simulink model "Gateway"  (R2025b)
settings: Solver=FixedStepDiscrete  StartTime=0.0  StopTime=inf  FixedStep=0.01  RelTol=1e-3
StartFcn:
  | qgcMavlinkGatewayVectorStep('reset');
StopFcn:
  | qgcMavlinkGatewayVectorStep('release');
undefined symbols (not defined in the file): CMD_MISSION_CRUISE_SPEED, CMD_MISSION_MAX_ACCELERATION, CMD_MISSION_MAX_JERK
settings Model: DataDictionary=CommandDict.sldd  Creator=89447  LastModifiedBy=89447
settings OptimizationCC: DefaultParameterBehavior=Inlined  EnhancedBackFolding=on  PassReuseOutputArgsAs=Individual arguments  ZeroExternalMemoryAtStartup=off  ZeroInternalMemoryAtStartup=off  MaxStackSize=64  OptimizeBlockOrder=speed  DifferentSizesBufferReuse=on  OptimizationCustomize=off  EfficientTunableParamExpr=on
settings HardwareCC: ProdBitPerLong=64.0  ProdHWDeviceType=Intel->x86-64 (Linux 64)  TargetBitPerLong=64.0  TargetBitPerPointer=64.0  TargetBitPerSizeT=64.0  TargetBitPerPtrDiffT=64.0  TargetLargestAtomicFloat=Float  TargetIntDivRoundTo=Zero  TargetEndianess=LittleEndian  TargetWordSize=64.0  TargetHWDeviceType=Intel->x86-64 (Linux 64)  ProdEqTarget=off
settings ModelReferenceCC: ModelReferenceNumInstancesAllowed=Single
settings SFSimCC: MATLABDynamicMemAlloc=off
settings RTWCC: SystemTargetFile=ert.tlc  HardwareBoard=Robot Operating System 2 (ROS 2)  TLCOptions="-aInlineSetEventsForThisBaseRateFcn=TLC_FALSE -aSuppressMultiTaskScheduler=TLC_FALSE  -aRateBasedStepFcn=0"  TemplateMakefile=ert_default_tmf  Toolchain=Colcon Tools  TargetLang=C++  Description=Embedded Coder
settings CodeAppCC: ForceParamTrailComments=on  IgnoreCustomStorageClasses=off  OperatorAnnotations=on  SimulinkDataObjDesc=on  SFDataObjDesc=on  InsertBlockDesc=on
settings ERTTargetCC: ExtModeTransport=2.0  ExtModeStaticAlloc=on  ExtModeMexFile=ext_xcp  ExtModeIntrfLevel=Level2 - Open  ERTCustomFileTemplate=example_file_process.tlc  TargetLangStandard=C++11 (ISO)  SubcomponentCodeInterfacePackaging=Nonreusable function  SupportContinuousTime=on

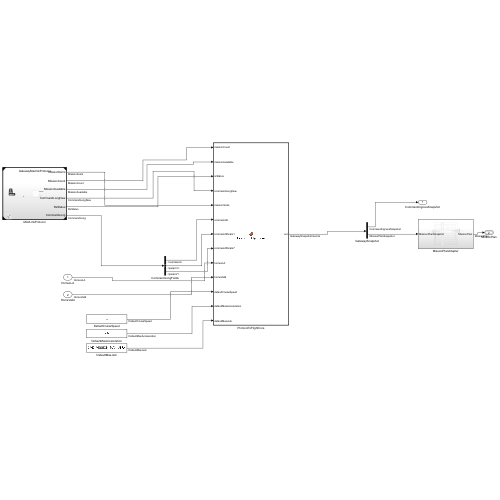
[thumbnail: Simulink's stored preview of the top-level diagram]
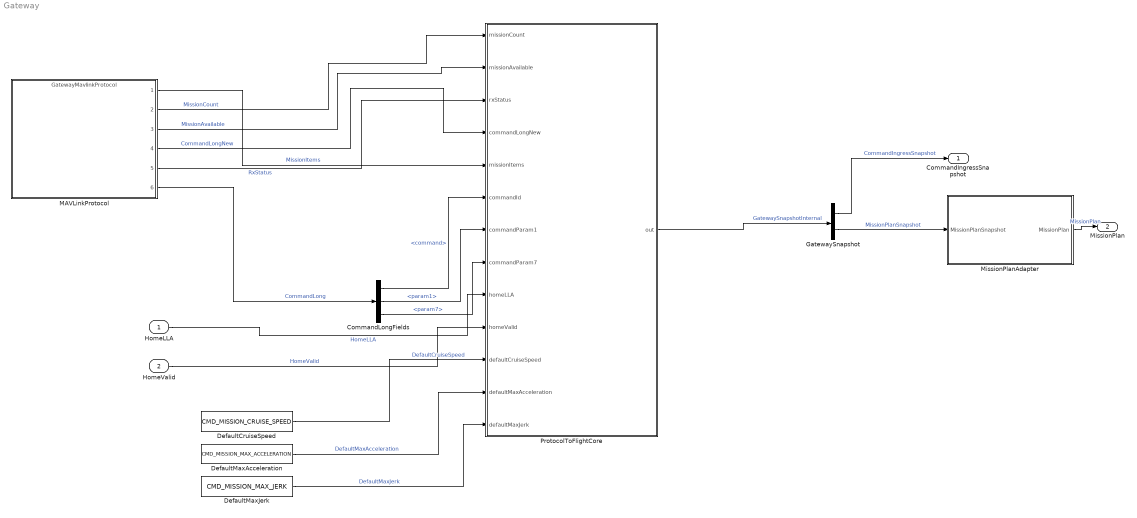
== system Gateway ==
  HomeLLA : Inport  OutDataTypeStr=single  PortDimensions=3
  HomeValid : Inport  Port=2  OutDataTypeStr=boolean  PortDimensions=1
  CommandLongFields : BusSelector  OutputSignals=Payload.command,Payload.param1,Payload.param7
  DefaultCruiseSpeed : Constant  Value=CMD_MISSION_CRUISE_SPEED  OutDataTypeStr=single
  DefaultMaxAcceleration : Constant  Value=CMD_MISSION_MAX_ACCELERATION  OutDataTypeStr=single
  DefaultMaxJerk : Constant  Value=CMD_MISSION_MAX_JERK  OutDataTypeStr=single
  GatewaySnapshot : Demux  Outputs=[17 123]
  MAVLinkProtocol : ModelReference  ModelNameDialog=GatewayMavlinkProtocol  ModelReferenceVersion=10.22
  MissionPlanAdapter : Subsystem
  ProtocolToFlightCore : MATLAB Function  TreatAsAtomicUnit=on
  CommandIngressSnapshot : Outport
  MissionPlan : Outport  Port=2  OutDataTypeStr=Bus: MissionPlanBus
  wires:
  GatewaySnapshot/1 -> CommandIngressSnapshot/1  "CommandIngressSnapshot"
  GatewaySnapshot/2 -> MissionPlanAdapter/1(MissionPlanSnapshot)  "MissionPlanSnapshot"
  MissionPlanAdapter/1(MissionPlan) -> MissionPlan/1  "MissionPlan"
  MAVLinkProtocol/2 -> ProtocolToFlightCore/1(missionCount)  "MissionCount"
  MAVLinkProtocol/3 -> ProtocolToFlightCore/2(missionAvailable)  "MissionAvailable"
  MAVLinkProtocol/4 -> ProtocolToFlightCore/4(commandLongNew)  "CommandLongNew"
  CommandLongFields/1 -> ProtocolToFlightCore/6(commandId)  "<command>"
  CommandLongFields/2 -> ProtocolToFlightCore/7(commandParam1)  "<param1>"
  CommandLongFields/3 -> ProtocolToFlightCore/8(commandParam7)  "<param7>"
  HomeLLA/1 -> ProtocolToFlightCore/9(homeLLA)  "HomeLLA"
  HomeValid/1 -> ProtocolToFlightCore/10(homeValid)  "HomeValid"
  DefaultCruiseSpeed/1 -> ProtocolToFlightCore/11(defaultCruiseSpeed)  "DefaultCruiseSpeed"
  DefaultMaxAcceleration/1 -> ProtocolToFlightCore/12(defaultMaxAcceleration)  "DefaultMaxAcceleration"
  DefaultMaxJerk/1 -> ProtocolToFlightCore/13(defaultMaxJerk)  "DefaultMaxJerk"
  ProtocolToFlightCore/1(out) -> GatewaySnapshot/1  "GatewaySnapshotInternal"
  MAVLinkProtocol/5 -> ProtocolToFlightCore/3(rxStatus)  "RxStatus"
  MAVLinkProtocol/6 -> CommandLongFields/1  "CommandLong"
  MAVLinkProtocol/1 -> ProtocolToFlightCore/5(missionItems)  "MissionItems"

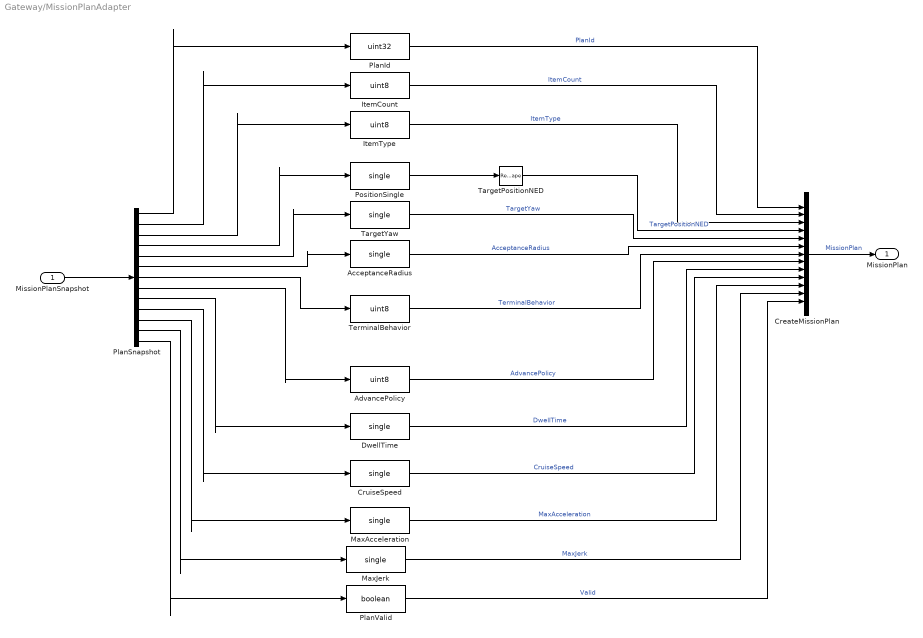
== system Gateway/MissionPlanAdapter ==
  MissionPlanSnapshot : Inport  OutDataTypeStr=double  PortDimensions=123
  AcceptanceRadius : DataTypeConversion  OutDataTypeStr=single
  AdvancePolicy : DataTypeConversion  OutDataTypeStr=uint8
  CreateMissionPlan : BusCreator  Inputs=13  OutDataTypeStr=Bus: MissionPlanBus  NonVirtualBus=on
  CruiseSpeed : DataTypeConversion  OutDataTypeStr=single
  DwellTime : DataTypeConversion  OutDataTypeStr=single
  ItemCount : DataTypeConversion  OutDataTypeStr=uint8
  ItemType : DataTypeConversion  OutDataTypeStr=uint8
  MaxAcceleration : DataTypeConversion  OutDataTypeStr=single
  MaxJerk : DataTypeConversion  OutDataTypeStr=single
  PlanId : DataTypeConversion  OutDataTypeStr=uint32
  PlanSnapshot : Demux  Outputs=[1 1 10 30 10 10 10 10 10 10 10 10 1]
  PlanValid : DataTypeConversion  OutDataTypeStr=boolean
  PositionSingle : DataTypeConversion  OutDataTypeStr=single
  TargetPositionNED : Reshape  OutputDimensionality=Customize  OutputDimensions=[10 3]
  TargetYaw : DataTypeConversion  OutDataTypeStr=single
  TerminalBehavior : DataTypeConversion  OutDataTypeStr=uint8
  MissionPlan : Outport  OutDataTypeStr=Bus: MissionPlanBus
  wires:
  MissionPlanSnapshot/1 -> PlanSnapshot/1
  PlanSnapshot/1 -> PlanId/1
  PlanSnapshot/2 -> ItemCount/1
  PlanSnapshot/3 -> ItemType/1
  PlanSnapshot/4 -> PositionSingle/1
  PositionSingle/1 -> TargetPositionNED/1
  PlanSnapshot/5 -> TargetYaw/1
  PlanSnapshot/6 -> AcceptanceRadius/1
  PlanSnapshot/7 -> TerminalBehavior/1
  PlanSnapshot/8 -> AdvancePolicy/1
  PlanId/1 -> CreateMissionPlan/1  "PlanId"
  ItemCount/1 -> CreateMissionPlan/2  "ItemCount"
  ItemType/1 -> CreateMissionPlan/3  "ItemType"
  TargetPositionNED/1 -> CreateMissionPlan/4  "TargetPositionNED"
  TargetYaw/1 -> CreateMissionPlan/5  "TargetYaw"
  AcceptanceRadius/1 -> CreateMissionPlan/6  "AcceptanceRadius"
  TerminalBehavior/1 -> CreateMissionPlan/7  "TerminalBehavior"
  AdvancePolicy/1 -> CreateMissionPlan/8  "AdvancePolicy"
  CreateMissionPlan/1 -> MissionPlan/1  "MissionPlan"
  PlanSnapshot/13 -> PlanValid/1
  PlanValid/1 -> CreateMissionPlan/13  "Valid"
  PlanSnapshot/9 -> DwellTime/1
  DwellTime/1 -> CreateMissionPlan/9  "DwellTime"
  PlanSnapshot/10 -> CruiseSpeed/1
  CruiseSpeed/1 -> CreateMissionPlan/10  "CruiseSpeed"
  PlanSnapshot/11 -> MaxAcceleration/1
  MaxAcceleration/1 -> CreateMissionPlan/11  "MaxAcceleration"
  PlanSnapshot/12 -> MaxJerk/1
  MaxJerk/1 -> CreateMissionPlan/12  "MaxJerk"

== matlab function Gateway/ProtocolToFlightCore ==
  data: missionCount input; out output; missionAvailable input; rxStatus input; commandLongNew input; missionItems input; commandId input; commandParam1 input; commandParam7 input; homeLLA input; homeValid input; defaultCruiseSpeed input; defaultMaxAcceleration input; defaultMaxJerk input
function out = ProtocolToFlightCore(missionCount, missionAvailable, rxStatus, commandLongNew, missionItems, commandId, commandParam1, commandParam7, homeLLA, homeValid, defaultCruiseSpeed, defaultMaxAcceleration, defaultMaxJerk)
%#codegen
persistent planId lastMissionAvailable rxSequence requestId nowSec lastRxTime linkAge
persistent commanderRequestType commanderRequestValid
persistent missionAction missionRequestValid missionRequestPlanId missionTargetAltitude
if isempty(planId)
    planId = uint32(0);
    lastMissionAvailable = false;
    rxSequence = uint32(0);
    requestId = uint32(0);
    nowSec = single(0);
    lastRxTime = single(0);
    linkAge = single(1000);
    commanderRequestType = uint8(0);
    commanderRequestValid = false;
    missionAction = uint8(0);
    missionRequestValid = false;
    missionRequestPlanId = uint32(0);
    missionTargetAltitude = single(0);
end
out = zeros(1,140);
nowSec = nowSec + single(0.1);
if rxStatus > 0
    rxSequence = rxSequence + uint32(1);
    lastRxTime = nowSec;
    linkAge = single(0);
else
    linkAge = linkAge + single(0.1);
end
connected = linkAge <= single(3.0);
if missionAvailable && ~lastMissionAvailable
    planId = planId + uint32(1);
end
lastMissionAvailable = missionAvailable;
if commandLongNew
    requestId = requestId + uint32(1);
    commanderRequestType = uint8(0);
    commanderRequestValid = false;
    missionAction = uint8(0);
    missionRequestValid = false;
    missionRequestPlanId = uint32(0);
    missionTargetAltitude = single(0);
    command = uint16(commandId);
    if command == uint16(400)
        if commandParam1 >= single(0.5)
            commanderRequestType = uint8(3);
        else
            commanderRequestType = uint8(4);
        end
        commanderRequestValid = true;
    elseif command == uint16(185) && commandParam1 >= single(0.5)
        commanderRequestType = uint8(5);
        commanderRequestValid = true;
    elseif command == uint16(300)
        missionAction = uint8(1);
        missionRequestPlanId = planId;
        missionRequestValid = true;
    elseif command == uint16(193)
        if commandParam1 >= single(0.5)
            missionAction = uint8(3);
        else
            missionAction = uint8(2);
        end
        missionRequestPlanId = planId;
        missionRequestValid = true;
    elseif command == uint16(22)
        missionAction = uint8(6);
        missionTargetAltitude = single(commandParam7);
        missionRequestPlanId = planId;
        missionRequestValid = true;
    elseif command == uint16(21)
        missionAction = uint8(7);
        missionTargetAltitude = single(0);
        missionRequestPlanId = planId;
        missionRequestValid = true;
    end
end
out(1) = double(connected);
out(2) = 255;
out(3) = double(rxSequence);
out(4) = double(lastRxTime);
out(5) = double(connected);
out(6) = double(connected);
out(7) = double(requestId);
out(8) = 255;
out(9) = double(commanderRequestType);
out(10) = double(commanderRequestValid);
out(11) = double(requestId);
out(12) = 255;
out(13) = double(missionRequestPlanId);
out(14) = double(missionAction);
out(15) = 0;
out(16) = double(missionTargetAltitude);
out(17) = double(missionRequestValid);
itemType = zeros(1,10,'uint8');
north = zeros(1,10,'single');
east = zeros(1,10,'single');
down = zeros(1,10,'single');
yaw = zeros(1,10,'single');
acceptance = zeros(1,10,'single');
terminal = zeros(1,10,'uint8');
advance = zeros(1,10,'uint8');
dwell = zeros(1,10,'single');
speed = zeros(1,10,'single');
maxAccel = zeros(1,10,'single');
maxJerk = zeros(1,10,'single');
routeCount = uint8(0);
planValid = false;
currentSpeed = single(defaultCruiseSpeed);
count = min(uint16(missionCount),uint16(10));
if missionAvailable && homeValid && count >= uint16(1) && currentSpeed > single(0) && defaultMaxAcceleration > single(0) && defaultMaxJerk > single(0)
    valid = true;
    homeLat = double(homeLLA(1));
    homeLon = double(homeLLA(2));
    homeAlt = double(homeLLA(3));
    for k = 1:10
        if k > double(count)
            break
        end
        cmd = uint16(missionItems(k).command);
        if cmd == uint16(178)
            if isfinite(double(missionItems(k).param2)) && missionItems(k).param2 > single(0)
                currentSpeed = single(missionItems(k).param2);
            else
                valid = false;
            end
            continue
        end
        if cmd == uint16(22)
            kind = uint8(1);
        elseif cmd == uint16(16)
            kind = uint8(2);
        elseif cmd == uint16(21)
            kind = uint8(3);
        else
            valid = false;
            kind = uint8(0);
        end
        frame = uint8(missionItems(k).frame);
        lat = double(missionItems(k).x)*1.0e-7;
        lon = double(missionItems(k).y)*1.0e-7;
        alt = double(missionItems(k).z);
        if frame == uint8(6)
            alt = homeAlt + alt;
        elseif frame ~= uint8(5)
            valid = false;
        end
        radius = single(missionItems(k).param2);
        if ~isfinite(lat) || ~isfinite(lon) || ~isfinite(alt) || abs(lat) > 90 || abs(lon) > 180 || ~isfinite(double(radius)) || radius <= single(0)
            valid = false;
        end
        if routeCount >= uint8(10)
            valid = false;
        else
            routeCount = routeCount + uint8(1);
            idx = double(routeCount);
            dLat = (lat-homeLat)*(pi/180);
            dLon = (lon-homeLon)*(pi/180);
            north(idx) = single(6378137.0*dLat);
            east(idx) = single(6378137.0*cos(homeLat*pi/180)*dLon);
            down(idx) = single(homeAlt-alt);
            itemType(idx) = kind;
            yawDeg = double(missionItems(k).param4);
            if ~isfinite(yawDeg)
                yawDeg = 0;
            end
            yaw(idx) = single(yawDeg*pi/180);
            acceptance(idx) = radius;
            terminal(idx) = uint8(0);
            advance(idx) = uint8(missionItems(k).autocontinue ~= 0);
            dwell(idx) = single(0);
            speed(idx) = currentSpeed;
            maxAccel(idx) = single(defaultMaxAcceleration);
            maxJerk(idx) = single(defaultMaxJerk);
        end
    end
    planValid = valid && routeCount >= uint8(1);
end
out(18) = double(planId);
out(19) = double(routeCount);
out(20:29) = double(itemType);
out(30:39) = double(north);
out(40:49) = double(east);
out(50:59) = double(down);
out(60:69) = double(yaw);
out(70:79) = double(acceptance);
out(80:89) = double(terminal);
out(90:99) = double(advance);
out(100:109) = double(dwell);
out(110:119) = double(speed);
out(120:129) = double(maxAccel);
out(130:139) = double(maxJerk);
out(140) = double(planValid);
